simulink model "LinearSimulationMess"  (R2017a)
settings: Solver=VariableStepAuto  StartTime=0.0  StopTime=10  MaxStep=1e-5  RelTol=1e-5
libraries: simulink x3
settings Model: Creator=khrom  LastModifiedBy=khrom

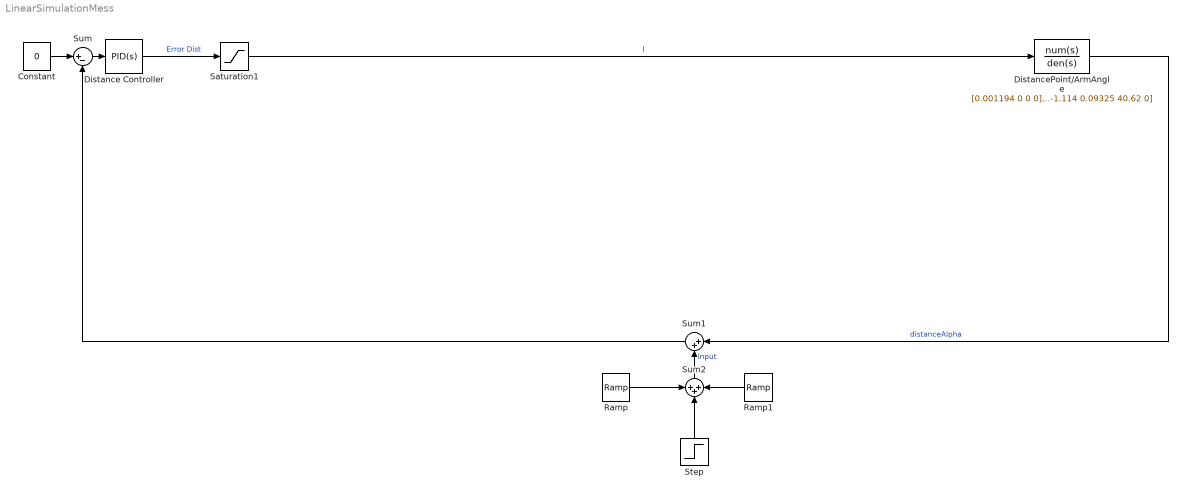
== system LinearSimulationMess ==
  Constant : Constant  Value=0
  Distance Controller : simulink/Continuous/PID Controller  Controller=PID  TimeDomain=Continuous-time  SampleTime=-1  IntegratorMethod=Forward Euler  FilterMethod=Forward Euler  Form=Parallel  UseFilter=off  ControllerParametersSource=internal  P=1.12e03  I=0.001*1.12e3  D=0.005*1.12e3  N=100  InitialConditionSource=internal  InitialConditionForIntegrator=0  InitialConditionForFilter=0  ExternalReset=none  LimitOutput=off  UpperSaturationLimit=inf  LowerSaturationLimit=-inf  LinearizeAsGain=off  AntiWindupMode=none  Kb=1  TrackingMode=off  Kt=1  PParamMin=[]  PParamMax=[]  IParamMin=[]  IParamMax=[]  DParamMin=[]  DParamMax=[]  NParamMin=[]  NParamMax=[]  KbParamMin=[]  KbParamMax=[]  KtParamMin=[]  KtParamMax=[]  POutMin=[]  POutMax=[]  IOutMin=[]  IOutMax=[]  DOutMin=[]  DOutMax=[]  NOutMin=[]  NOutMax=[]  KbOutMin=[]  KbOutMax=[]  KtOutMin=[]  KtOutMax=[]  IntegratorOutMin=[]  IntegratorOutMax=[]  FilterOutMin=[]  FilterOutMax=[]  SumOutMin=[]  SumOutMax=[]  SumI1OutMin=[]  SumI1OutMax=[]  SumI2OutMin=[]  SumI2OutMax=[]  SumI3OutMin=[]  SumI3OutMax=[]  SumDOutMin=[]  SumDOutMax=[]  SaturationOutMin=[]  SaturationOutMax=[]  IntegratorContinuousStateAttributes=''  IntegratorStateMustResolveToSignalObject=off  IntegratorRTWStateStorageClass=Auto  FilterContinuousStateAttributes=''  FilterStateMustResolveToSignalObject=off  FilterRTWStateStorageClass=Auto  DifferentiatorICPrevScaledInput=0  DifferentiatorOutMin=[]  DifferentiatorOutMax=[]  InitialConditionSetting=State (most efficient)
  DistancePoint/ArmAngle : TransferFcn  Numerator=[0.001194 0 0 0]  Denominator=[0.0002338 -0.002537 -1.114 0.09325 40.62 0]
  Ramp : simulink/Sources/Ramp  slope=13*pi/180  start=0  X0=0
  Ramp1 : simulink/Sources/Ramp  slope=-13*pi/180  start=0.1  X0=0
  Saturation1 : Saturate  UpperLimit=11*0.8  LowerLimit=-11*0.8
  Step : Step  Time=0.1  After=-13*pi/180*0.1  SampleTime=0
  Sum : Sum  Inputs=|+-
  Sum1 : Sum  Inputs=|++
  Sum2 : Sum  Inputs=+++
  wires:
  Sum/1 -> Distance Controller/1
  Sum2/1 -> Sum1/2  "Input"
  Constant/1 -> Sum/1
  Ramp/1 -> Sum2/1
  Ramp1/1 -> Sum2/3
  Step/1 -> Sum2/2
  Sum1/1 -> Sum/2
  DistancePoint/ArmAngle/1 -> Sum1/1  "distanceAlpha"
  Distance Controller/1 -> Saturation1/1  "Error Dist"
  Saturation1/1 -> DistancePoint/ArmAngle/1  "I"
